simulink model "CTC_ARTICULAR1"  (R2015a)
settings: Solver=ode45  StartTime=0.0  StopTime=3  RelTol=1e-3
values from neighbouring files (symbols this model uses):
  KP1 = 100000    [INICIO.m]
  KP2 = 85000    [INICIO.m]
  KP3 = 70000    [INICIO.m]
  KP4 = 70000    [INICIO.m]
  KV1 = 360    [INICIO.m]
  KV2 = 280    [INICIO.m]
  KV3 = 120    [INICIO.m]
  KV4 = 120    [INICIO.m]
  Tem = 0.001    [INICIO.m]
undefined symbols (not defined in the file or in its folder): MDI
settings Model: CovHtmlReporting=off  Creator=ANDRES Y MARCELA  LastModifiedBy=Shadow
settings DataIOCC: SignalLoggingSaveFormat=ModelDataLogs
settings OptimizationCC: ExpressionDepthLimit=2147483647
settings DebuggingCC: UnderspecifiedInitializationDetection=Classic  MergeDetectMultiDrivingBlocksExec=none  SolverPrmCheckMsg=warning  FcnCallInpInsideContextMsg=EnableAllAsWarning  StateNameClashWarn=warning
settings GRTTargetCC: CombineOutputUpdateFcns=off  GRTInterface=on

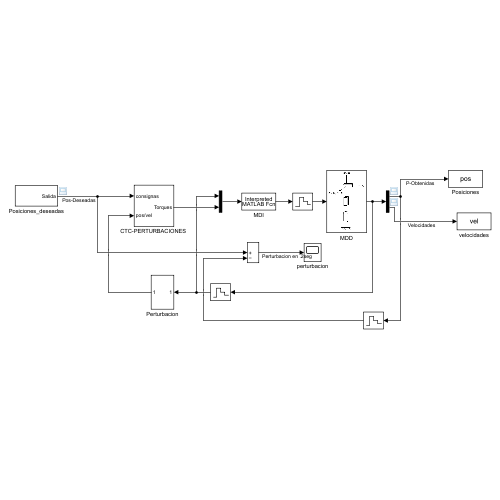
[thumbnail: Simulink's stored preview of the top-level diagram]
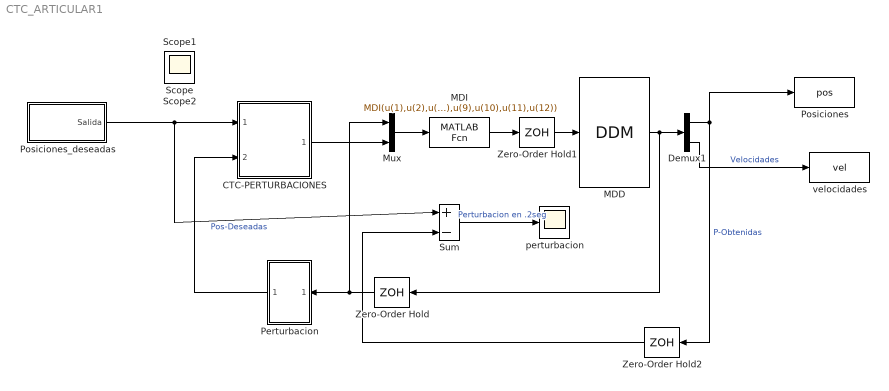
== system CTC_ARTICULAR1 ==
  "CTC-PERTURBACIONES " : Subsystem
  Demux1 : Demux  Outputs=2
  MDD : S-Function  FunctionName=DDM  Parameters=QI  SFunctionDeploymentMode=off  EnableBusSupport=off
      mask Display: image(imread('robot.jpg'))
  MDI : MATLABFcn  MATLABFcn=MDI(u(1),u(2),u(3),u(4),u(5),u(6),u(7),u(8),u(9),u(10),u(11),u(12))  OutputDimensions=4
  Mux : Mux  Inputs=2
  Perturbacion : Subsystem
  Posiciones : ToWorkspace  VariableName=pos  SampleTime=-1
  Posiciones_deseadas : Subsystem
  Sum : Sum  Inputs=|+-
  Zero-Order Hold : ZeroOrderHold  SampleTime=Tem
  Zero-Order Hold1 : ZeroOrderHold  SampleTime=Tem
  Zero-Order Hold2 : ZeroOrderHold  SampleTime=Tem
  perturbacion : Scope
      settings: TimeRange=auto  LimitDataPoints=on  MaxDataPoints=5000  SaveToWorkspace=off  SaveName=ScopeData  YMin=-0.23665  YMax=0.37816  SampleTime=-1
  velocidades : ToWorkspace  VariableName=vel  SampleTime=-1
  Scope : Scope
      settings: TimeRange=auto  MaxDataPoints=5000  SaveToWorkspace=off  YMin=-0.18752  YMax=1.68765  SampleTime=-1
  Scope1 : Scope
      settings: TimeRange=auto  MaxDataPoints=5000  SaveToWorkspace=off  SaveName=ScopeData2  YMin=-33.20776  YMax=49.53803  SampleTime=-1
  Scope2 : Scope
      settings: TimeRange=auto  MaxDataPoints=5000  SaveToWorkspace=off  SaveName=ScopeData3  YMin=-0.1875  YMax=1.6875  SampleTime=-1
  wires:
  Perturbacion/1(Out1) -> "CTC-PERTURBACIONES "/2(pos/vel)
  Zero-Order Hold2/1 -> Sum/2
  Zero-Order Hold/1 -> Mux/1, Perturbacion/1(In1)
  Demux1/2 -> velocidades/1  "Velocidades"
  Mux/1 -> MDI/1
  Sum/1 -> perturbacion/1  "Perturbacion en .2seg"
  "CTC-PERTURBACIONES "/1(Torques) -> Mux/2
  Zero-Order Hold1/1 -> MDD/1
  Demux1/1 -> Posiciones/1, Zero-Order Hold2/1  "P-Obtenidas"
  MDI/1 -> Zero-Order Hold1/1
  Posiciones_deseadas/1(Salida) -> "CTC-PERTURBACIONES "/1(consignas), Sum/1  "Pos-Deseadas"
  MDD/1 -> Demux1/1, Zero-Order Hold/1

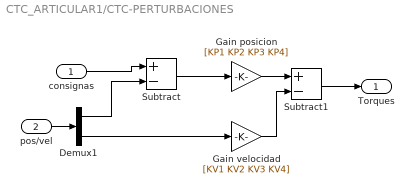
== system CTC_ARTICULAR1/CTC-PERTURBACIONES  ==
  consignas : Inport
  pos/vel : Inport  Port=2
  Demux1 : Demux  Outputs=2
  Gain posicion : Gain  Gain=[KP1 KP2 KP3 KP4]
  Gain velocidad : Gain  Gain=[KV1 KV2 KV3 KV4]
  Subtract : Sum  Inputs=+-
  Subtract1 : Sum  Inputs=+-
  Torques : Outport
  wires:
  Subtract/1 -> Gain posicion/1
  Gain posicion/1 -> Subtract1/1
  Gain velocidad/1 -> Subtract1/2
  Demux1/1 -> Subtract/2
  Demux1/2 -> Gain velocidad/1
  consignas/1 -> Subtract/1
  pos/vel/1 -> Demux1/1
  Subtract1/1 -> Torques/1

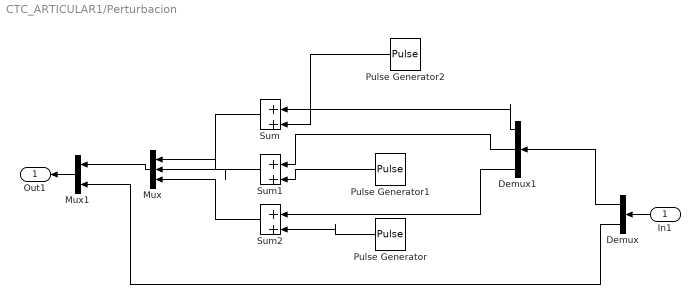
== system CTC_ARTICULAR1/Perturbacion ==
  In1 : Inport
  Demux : Demux  Outputs=2
  Demux1 : Demux  Outputs=3
  Mux : Mux  Inputs=3
  Mux1 : Mux  Inputs=2
  Pulse Generator : DiscretePulseGenerator  PulseType=Time based  Amplitude=0.2  Period=10  PulseWidth=0.1  PhaseDelay=0.3
  Pulse Generator1 : DiscretePulseGenerator  PulseType=Time based  Amplitude=0.2  Period=10  PulseWidth=0.1  PhaseDelay=0.3
  Pulse Generator2 : DiscretePulseGenerator  PulseType=Time based  Amplitude=0.2  Period=10  PulseWidth=0.1  PhaseDelay=0.3
  Sum : Sum  Inputs=|++
  Sum1 : Sum  Inputs=|++
  Sum2 : Sum  Inputs=|++
  Out1 : Outport
  wires:
  In1/1 -> Demux/1
  Mux1/1 -> Out1/1
  Demux/2 -> Mux1/2
  Mux/1 -> Mux1/1
  Sum2/1 -> Mux/3
  Sum1/1 -> Mux/2
  Sum/1 -> Mux/1
  Pulse Generator/1 -> Sum2/2
  Demux1/3 -> Sum2/1
  Demux1/2 -> Sum1/1
  Pulse Generator1/1 -> Sum1/2
  Pulse Generator2/1 -> Sum/2
  Demux1/1 -> Sum/1
  Demux/1 -> Demux1/1

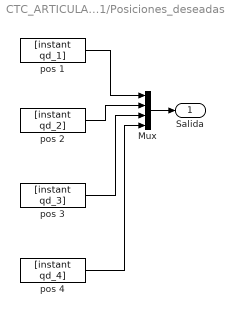
== system CTC_ARTICULAR1/Posiciones_deseadas ==
  Mux : Mux
  pos 1 : FromWorkspace  VariableName=[instant qd_1]  SampleTime=Tem  ZeroCross=off
  pos 2 : FromWorkspace  VariableName=[instant qd_2]  SampleTime=Tem  ZeroCross=off
  pos 3 : FromWorkspace  VariableName=[instant qd_3]  SampleTime=Tem  ZeroCross=off
  pos 4 : FromWorkspace  VariableName=[instant qd_4]  SampleTime=Tem  ZeroCross=off
  Salida : Outport
  wires:
  pos 1/1 -> Mux/1
  pos 2/1 -> Mux/2
  pos 3/1 -> Mux/3
  Mux/1 -> Salida/1
  pos 4/1 -> Mux/4
